simulink model "FPGA_Modem_Sim"  (R2020a)
settings: Solver=VariableStepAuto  StartTime=0.0  StopTime=stop_time  RelTol=1e-3
values from neighbouring files (symbols this model uses):
  A = 1    [FPGA_Modem_Main.m]    (also in Mod_Output.m = 8191)
  alpha = 0.8    [FPGA_Modem_Main.m]
  Bits_Num = 8    [FPGA_Modem_Main.m]
  Dec_factor_1 = 30    [FPGA_Modem_Main.m]
  Fc = 33.25e6    (= 33250000)    [FPGA_Modem_Main.m]
  FFT_Length = 512    [FPGA_Modem_Main.m]
  fix_FL = 8    [FPGA_Modem_Main.m]
  fix_WL = 10    [FPGA_Modem_Main.m]
  Frame_Size = 64    [FPGA_Modem_Main.m]
  Fs = 150e6    (= 150000000)    [FPGA_Modem_Main.m]
  jitter = 5*1e-12    (= 5e-12)    [FPGA_Modem_Main.m]
  T_sym = 1e-6    (= 1e-06)    [FPGA_Modem_Main.m]
undefined symbols (not defined in the file or in its folder): magnitude
libraries: dspsigops x1, msbAdcFoundation x1, commdigbbndpm3 x1, commrandsrc3 x1, dspmlti4 x1, dsphdlxfrm x1, dspsrcs4 x1, dspmathops x1
settings Model: Creator=chuma  LastModifiedBy=chuma
settings OptimizationCC: BlockReduction=off  ConditionallyExecuteInputs=off  DefaultParameterBehavior=Inlined
settings DebuggingCC: AlgebraicLoopMsg=error
settings HardwareCC: ProdBitPerPointer=32  ProdBitPerSizeT=32  ProdBitPerPtrDiffT=32  ProdLargestAtomicFloat=None  ProdIntDivRoundTo=Undefined  ProdEndianess=Unspecified  ProdWordSize=32  ProdHWDeviceType=ASIC/FPGA->ASIC/FPGA  TargetBitPerPointer=64  TargetBitPerSizeT=64  TargetBitPerPtrDiffT=64  TargetLongLongMode=on  TargetIntDivRoundTo=Zero  TargetEndianess=LittleEndian  TargetWordSize=64  TargetHWDeviceType=Custom Processor->MATLAB Host Computer  ProdEqTarget=off

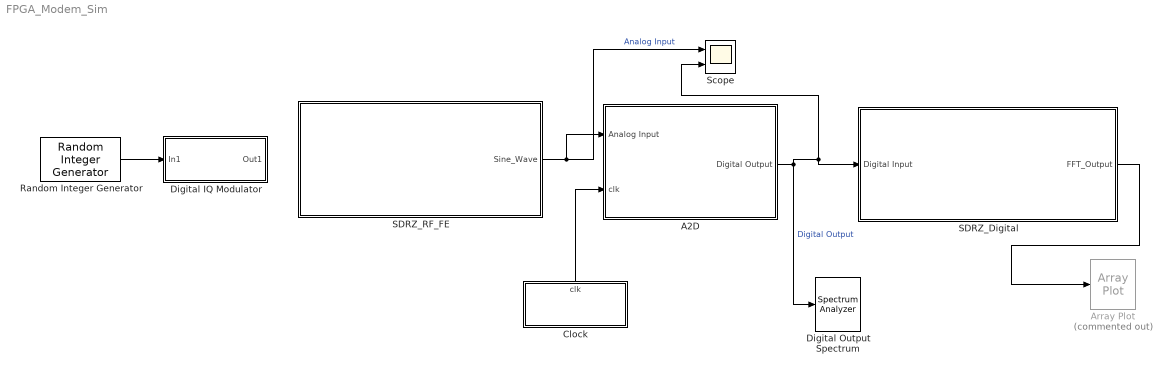
== system FPGA_Modem_Sim ==
  A2D : Subsystem
  Array Plot : ArrayPlot  Commented=on
  Clock : Subsystem
      settings: PortSchema="{\"entries\":[{\"content\":{\"sides\":[{\"content\":{\"connectorIds\":[]},\"type\":\"ConnectorPlacement.EquallySpacedRectSide\",\"uuid\":\"1fa5756f-f9d0-4514-88dd-c692581742d9\"},{\"content\":{\"connectorIds\":[],\"side\":\"RIGHT\"},\"type\":\"ConnectorPlacement.EquallySpacedRectSide\",\"uuid\":\"88e746c8-6142-4f87-ba53-01cde611927c\"},{\"content\":{\"connectorIds\":[\"Out1\"],\"side\":\"TOP\"},\"type\":\"ConnectorPlacement.EquallySpacedRectSide\",\"uuid\":\"b710edb4-a381-49b0-b2f3-0f4f3a2b2b74\"}]},\"type\":\"ConnectorPlacement.EquallySpacedConnector\",\"uuid\":\"ae7b1141-0622-4913-88c4-b2686b95aab4\"}],\"packageUris\":[\"http://schema.mathworks.com/mf0/Connector/19700101\"],\"version\":\"1.0\"}"
  Digital IQ Modulator : Subsystem
  Digital Output Spectrum : SpectrumAnalyzer
  Random Integer Generator : commrandsrc3/Random Integer Generator  SetSize=Mod_Order  SeedSource=Auto  Seed=37  SampleTime=T_sym  SamplesPerFrame=Frame_Size  OutputDataType=double  SimulateUsing=Interpreted execution
  SDRZ_Digital : Subsystem
  "SDRZ_RF_FE " : Subsystem
  Scope : Scope  NumInputPorts=2
  wires:
  SDRZ_Digital/1(FFT_Output) -> Array Plot/1
  "SDRZ_RF_FE "/1("Sine_Wave ") -> Scope/1, A2D/1(Analog Input)  "Analog Input"
  Clock/1(clk) -> A2D/2(clk)
  A2D/1(Digital Output) -> Scope/2, SDRZ_Digital/1(Digital Input), Digital Output Spectrum/1  "Digital Output"
  Random Integer Generator/1 -> Digital IQ Modulator/1(In1)

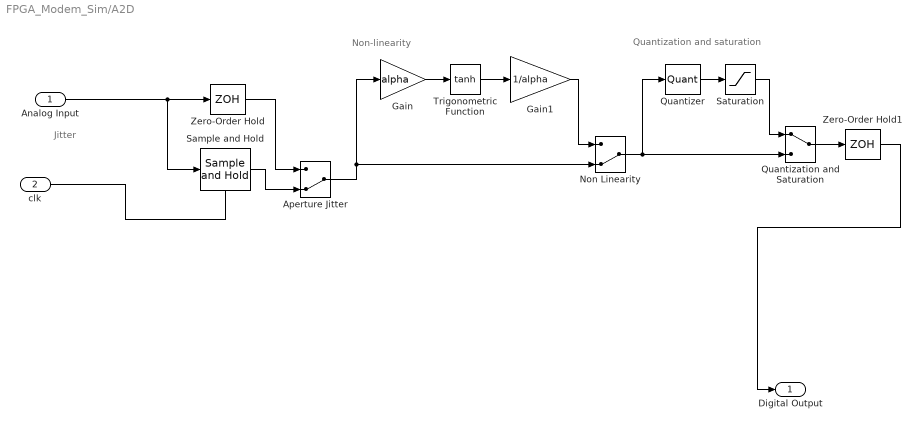
== system FPGA_Modem_Sim/A2D ==
  note: Non-linearity
  note: Jitter
  note: Quantization and saturation
  Analog Input : Inport
  clk : Inport  Port=2
  Aperture Jitter : ManualSwitch  CurrentSetting=0
  Gain : Gain  Gain=alpha
  Gain1 : Gain  Gain=1/alpha
  Non Linearity : ManualSwitch  CurrentSetting=0
  Quantization and Saturation : ManualSwitch
  Quantizer : Quantizer  QuantizationInterval=2^-Bits_Num
  Sample and Hold : dspsigops/Sample and Hold  trig=Rising edge  initCond=0  latchinput=off
  Saturation : Saturate  UpperLimit=1  LowerLimit=-1
  Trigonometric Function : Trigonometry  Operator=tanh
  Zero-Order Hold : ZeroOrderHold  SampleTime=1/Fs
  Zero-Order Hold1 : ZeroOrderHold  SampleTime=1/Fs
  Digital Output : Outport
  wires:
  Zero-Order Hold1/1 -> Digital Output/1
  Sample and Hold/1 -> Aperture Jitter/2
  Gain/1 -> Trigonometric Function/1
  Zero-Order Hold/1 -> Aperture Jitter/1
  Quantizer/1 -> Saturation/1
  Non Linearity/1 -> Quantization and Saturation/2, Quantizer/1
  Aperture Jitter/1 -> Gain/1, Non Linearity/2
  Saturation/1 -> Quantization and Saturation/1
  Gain1/1 -> Non Linearity/1
  Quantization and Saturation/1 -> Zero-Order Hold1/1
  Trigonometric Function/1 -> Gain1/1
  Analog Input/1 -> Sample and Hold/1, Zero-Order Hold/1
  clk/1 -> Sample and Hold/Trigger

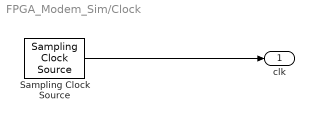
== system FPGA_Modem_Sim/Clock ==
  Sampling Clock Source : msbAdcFoundation/Sampling Clock Source  Freq=Fs  Min=-1  Max=1  RmsJitt=jitter*(1/Fs)  ExtraBuffer=off  NBuffer=5
      settings: SourceProductBaseCode=AM  SignalType=Square wave
  clk : Outport
  wires:
  Sampling Clock Source/1 -> clk/1

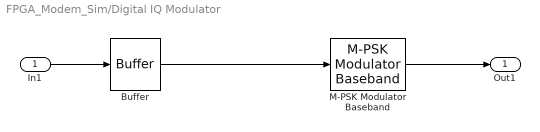
== system FPGA_Modem_Sim/Digital IQ Modulator ==
  In1 : Inport
  Buffer : Buffer  N=Frame_Size  OutputFrames=off
  M-PSK Modulator Baseband : commdigbbndpm3/M-PSK Modulator Baseband  M=Mod_Order  InType=Integer  Enc=Gray  Mapping=[0:7]  Ph=Phase_Offset  outDtype=Fixed-point  outWordLen=fix_WL  outUDDataType=sfix(16)  outFracLenMode=User-defined  outFracLen=fix_FL  outDataTypeStr=fixdt(1,fix_WL,fix_FL)  outLastDataTypeStr=fixdt(1,fix_WL,fix_FL)
  Out1 : Outport
  wires:
  In1/1 -> Buffer/1
  M-PSK Modulator Baseband/1 -> Out1/1
  Buffer/1 -> M-PSK Modulator Baseband/1

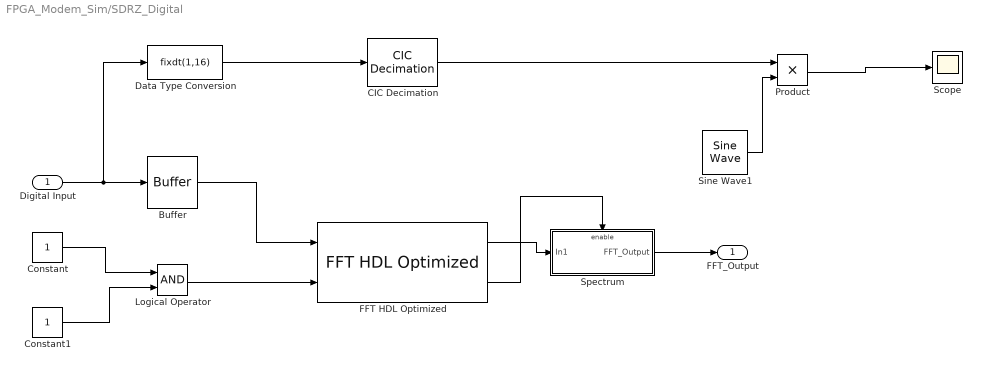
== system FPGA_Modem_Sim/SDRZ_Digital ==
  Digital Input : Inport
  Buffer : Buffer  N=Frame_Size  OutputFrames=off
  CIC Decimation : dspmlti4/CIC Decimation  filtFrom=Dialog parameters  filtobj=CICDECIM  ftype=Decimator  R=Dec_factor_1  M=1  N=2  filterInternals=Full precision  BPS=[16 16 16 16]  FLPS=0  outputWordLength=32  outputFracLength=0  launchFVT=off  framing=Maintain input frame rate  RateOptions=Allow multirate processing
      settings: SourceProductBaseCode=DS
  Constant : Constant
  Constant1 : Constant
  Data Type Conversion : DataTypeConversion  OutMin=[-1.5]  OutMax=[1.5]  OutDataTypeStr=fixdt(1,16)
  FFT HDL Optimized : dsphdlxfrm/FFT HDL Optimized  FFTLength=FFT_Length  Architecture=Streaming Radix 2^2  ComplexMultiplication=Use 4 multipliers and 2 adders  BitReversedOutput=off  BitReversedInput=off  Normalize=off  SimulateUsing=Code generation  RoundingMethod=Floor  ResetInputPort=off  StartOutputPort=off  EndOutputPort=off
      settings: SourceProductBaseCode=DS
  Logical Operator : Logic  AllPortsSameDT=off  OutDataTypeStr=boolean
  Product : Product
  Scope : Scope
  Sine Wave1 : dspsrcs4/Sine Wave  Amplitude=1  Frequency=Fc  Phase=pi/2  SampleMode=Discrete  OutComplex=Real  CompMethod=Trigonometric fcn  TableSize=Speed  SampleTime=Fc/Dec_factor_1  SamplesPerFrame=1  ResetState=Restart at time zero  OutputFrames=off  dataType=double  wordLen=16  udDataType=sfix(16)  fracBitsMode=Best precision  numFracBits=15  OutDataTypeStr=double  LastOutDataTypeStr=double
  Spectrum : Subsystem  TreatAsAtomicUnit=on
  FFT_Output : Outport
  wires:
  Digital Input/1 -> Data Type Conversion/1, Buffer/1
  Logical Operator/1 -> FFT HDL Optimized/2
  Constant/1 -> Logical Operator/1
  Constant1/1 -> Logical Operator/2
  FFT HDL Optimized/2 -> Spectrum/Enable
  FFT HDL Optimized/1 -> Spectrum/1(In1)
  Buffer/1 -> FFT HDL Optimized/1
  Spectrum/1(FFT_Output) -> FFT_Output/1
  Sine Wave1/1 -> Product/2
  CIC Decimation/1 -> Product/1
  Product/1 -> Scope/1
  Data Type Conversion/1 -> CIC Decimation/1

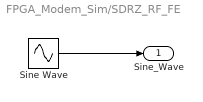
== system FPGA_Modem_Sim/SDRZ_RF_FE  ==
  Sine Wave : Sin  Amplitude=A  Frequency=2*pi*Fc  SampleTime=0
  "Sine_Wave " : Outport  VectorParamsAs1DForOutWhenUnconnected=off
  wires:
  Sine Wave/1 -> "Sine_Wave "/1

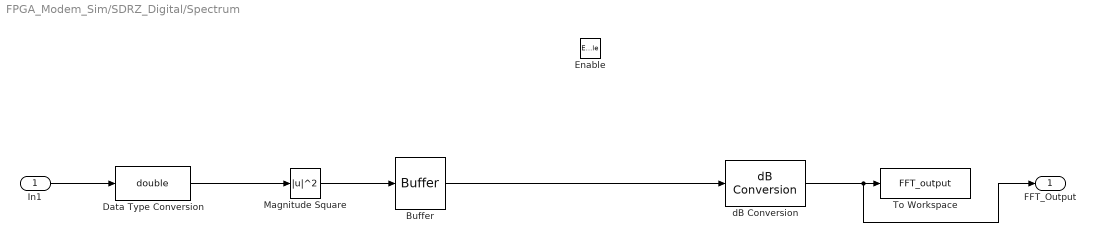
== system FPGA_Modem_Sim/SDRZ_Digital/Spectrum ==
  In1 : Inport
  Enable : EnablePort
  Buffer : Buffer  N=FFT_Length  OutputFrames=off
  Data Type Conversion : DataTypeConversion  OutDataTypeStr=double
  Magnitude Square : Math  Operator=magnitude^2  SignedPower=on  RndMeth=Zero  SaturateOnIntegerOverflow=on
  To Workspace : ToWorkspace  VariableName=FFT_output  SaveFormat=Structure With Time  SampleTime=-1
      settings: Save2DSignal=2-D array (concatenate along first dimension)
  dB Conversion : dspmathops/dB Conversion  dBtype=dB  intype=Amplitude  R=1  fuzz=on
  FFT_Output : Outport
  wires:
  In1/1 -> Data Type Conversion/1
  Buffer/1 -> dB Conversion/1
  Data Type Conversion/1 -> Magnitude Square/1
  dB Conversion/1 -> FFT_Output/1, To Workspace/1
  Magnitude Square/1 -> Buffer/1
